simulink library "motorAndLoadSFunLib"  (R2019a)
settings: Solver=ode45  StartTime=0.0  StopTime=10.0  RelTol=1e-3  EnableMultiTasking=on
settings Model: Creator=The MathWorks, Inc.  LastModifiedBy=The MathWorks, Inc.
settings DataIOCC: LimitDataPoints=on  SaveFormat=Array  ReturnWorkspaceOutputs=off
settings OptimizationCC: ExpressionDepthLimit=2147483647  LifeSpan=inf
settings DebuggingCC: UnderspecifiedInitializationDetection=Classic  MergeDetectMultiDrivingBlocksExec=none  SolverPrmCheckMsg=warning  AllowSymbolicDim=off  StateNameClashWarn=warning  SFUnexpectedBacktrackingDiag=warning  SFNoUnconditionalDefaultTransitionDiag=warning  SFExecutionAtInitializationDiag=none  ArithmeticOperatorsInVariantConditions=warning
settings HardwareCC: ProdBitPerPointer=32  ProdBitPerSizeT=32  ProdBitPerPtrDiffT=32  ProdLargestAtomicFloat=None  ProdIntDivRoundTo=Undefined  ProdEndianess=Unspecified  ProdWordSize=32  ProdHWDeviceType=32-bit Generic
settings ModelReferenceCC: PropagateSignalLabelsOutOfModel=off
settings SFSimCC: SimUseLocalCustomCode=off
settings RTWCC: RTWUseLocalCustomCode=off
settings CodeAppCC: StateflowObjectComments=on
settings GRTTargetCC: TargetLangStandard=C89/C90 (ANSI)  GeneratePreprocessorConditionals=Disable all
settings ConfigComp: CovMetricSettings=dw  CovHtmlReporting=on  CovSaveCumulativeToWorkspaceVar=on  CovSaveSingleToWorkspaceVar=on  CovExternalEMLEnable=off  CovSFcnEnable=off

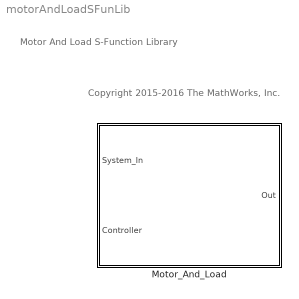
== system motorAndLoadSFunLib ==
  note: Motor And Load S-Function Library
  note: Copyright 2015-2016 The MathWorks, Inc.
  Motor_And_Load : Subsystem
      mask help:
      | This block is provided for users that do not have SimPowerSystems installed but still want to explore the system level simulation without changing motor and load parameter data.
      |
      | This block provides equiavelent functionality to the example library motorAndLoadSimPowerSystemsLib using the default data values included with this example. If you modify data associated with this example, they will NOT be reflected in this block.
      |
      | Please install SimPowerSystems to explore the effects of changing motor and load data including: pmsm, inverter, encoder, and adc values associated with this model.
      mask Display: image('focZynqMotorAndLoadMask.png');

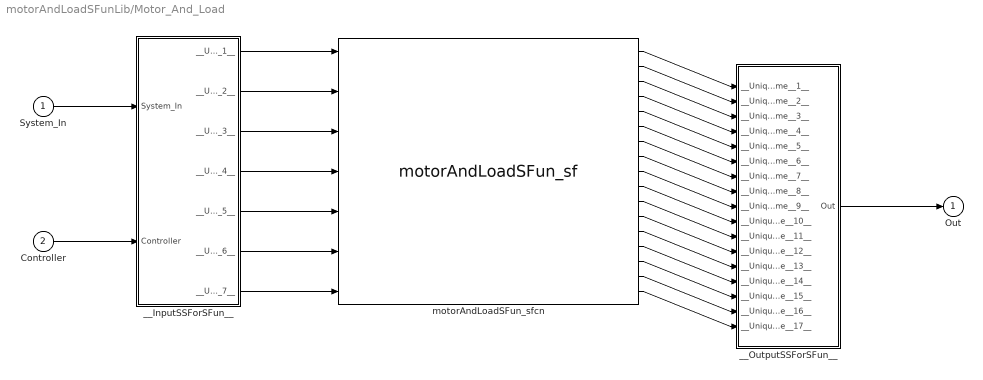
== system motorAndLoadSFunLib/Motor_And_Load ==
  System_In : Inport
  Controller : Inport  Port=2
  __InputSSForSFun__ : Subsystem
  __OutputSSForSFun__ : Subsystem
  motorAndLoadSFun_sfcn : S-Function  FunctionName=motorAndLoadSFun_sf  SFunctionModules=""  SFunctionDeploymentMode=off  EnableBusSupport=off  mask{rtw_sf_name=motorAndLoadSFun_sf, showVar=off}
      mask prompts: rtw_sf_name "Simulink:masks:GenSFuncName_MP"; showVar "Simulink:masks:GenSFuncShowModuleList_MP"
      mask help: Simulink:masks:GenSFuncDesc_MD
      mask init:
      | displist = '';
      | if ~strcmp(get_param(gcb, 'FunctionName'), rtw_sf_name);
      |   set_param(gcb, 'FunctionName', rtw_sf_name);
      | end
      | % Check if we are generating code
      | rtw_mode = false;
      | if strcmpi(get_param(bdroot(gcb),'SimulationStatus'),'Initializing')
      | 	rtw_mode = strcmpi(get_param(bdroot(gcb),'BuildingRTWCode'),'on') && ...
      | 		~strcmpi(get_param(bdroot(gcb),'TargetStyle'),'SimulationTarget');
      | end
      | if showVar || rtw_mode
      | 	if exist('rtwsfunc') == 2 | exist('rtwsfunc') == 6
      | 		tmplist = rtwsfunc(rtw_sf_name,gcb);
      | 		tmplist = DAStudio.message('Simulink:masks:GenSFuncListOfModules_IC', tmplist);
      | 	elseif showVar
      | 		tmplist1 = DAStudio.message('Simulink:masks:GenSFuncListOfModules_IC', '');
      |         tmplist2 = DAStudio.message('Simulink:masks:GenSFuncNotLicensed_IC');
      |         tmplist = [tmplist1 tmplist2];
      |  	end
      | end
      | if showVar
      |   displist = tmplist;
      | end
      settings: CopyFcn=|
      | if ~strcmp(get_param(gcb,'Linkstatus'),'none') && ...
      | ~strcmp(get_param(gcb,'Linkstatus'),'implicit')
      |   set_param(gcb,'LinkStatus','none');
      | end
      mask Help: eval('feval(''rtwprivate'',''rtwhelpview'',''rtw_sfcn_block'')');
      mask Display:
      | port_label('input',1,'motorOn');
      | port_label('input',2,'commandType');
      | port_label('input',3,'velocityCommand');
      | port_label('input',4,'dynoLoadDutyCycle');
      | port_label('input',5,'controllerMode');
      | port_label('input',6,'inverterEnable');
      | port_label('input',7,'pwmCompare');
      | port_label('output',1,'controllerModeb');
      | port_label('output',2,'inverterEnableb');
      | port_label('output',3,'pwmCompareb');
      | port_label('output',4,'phaseVoltage');
      | port_label('output',5,'phaseCurrentA');
      | port_label('output',6,'phaseCurrentB');
      | port_label('output',7,'phaseCurrentC');
      | port_label('output',8,'directCurrent');
      | port_label('output',9,'quadratureCurrent');
      | port_label('output',10,'electromagneticTorque');
      | port_label('output',11,'rotorPosition');
      | port_label('output',12,'electricalPosition');
      | port_label('output',13,'rotorVelocity');
      | port_label('output',14,'electricalVelocity');
      | port_label('output',15,'adcCount');
      | port_label('output',16,'encoderIndexFound');
      | port_label('output',17,'encoderCount');
  Out : Outport
  wires:
  __OutputSSForSFun__/1(Out) -> Out/1
  motorAndLoadSFun_sfcn/17 -> __OutputSSForSFun__/17(__UniqueInportName__17__)
  motorAndLoadSFun_sfcn/16 -> __OutputSSForSFun__/16(__UniqueInportName__16__)
  motorAndLoadSFun_sfcn/15 -> __OutputSSForSFun__/15(__UniqueInportName__15__)
  motorAndLoadSFun_sfcn/14 -> __OutputSSForSFun__/14(__UniqueInportName__14__)
  motorAndLoadSFun_sfcn/13 -> __OutputSSForSFun__/13(__UniqueInportName__13__)
  motorAndLoadSFun_sfcn/12 -> __OutputSSForSFun__/12(__UniqueInportName__12__)
  motorAndLoadSFun_sfcn/11 -> __OutputSSForSFun__/11(__UniqueInportName__11__)
  motorAndLoadSFun_sfcn/10 -> __OutputSSForSFun__/10(__UniqueInportName__10__)
  motorAndLoadSFun_sfcn/9 -> __OutputSSForSFun__/9(__UniqueInportName__9__)
  motorAndLoadSFun_sfcn/8 -> __OutputSSForSFun__/8(__UniqueInportName__8__)
  motorAndLoadSFun_sfcn/7 -> __OutputSSForSFun__/7(__UniqueInportName__7__)
  motorAndLoadSFun_sfcn/6 -> __OutputSSForSFun__/6(__UniqueInportName__6__)
  motorAndLoadSFun_sfcn/5 -> __OutputSSForSFun__/5(__UniqueInportName__5__)
  motorAndLoadSFun_sfcn/4 -> __OutputSSForSFun__/4(__UniqueInportName__4__)
  motorAndLoadSFun_sfcn/3 -> __OutputSSForSFun__/3(__UniqueInportName__3__)
  motorAndLoadSFun_sfcn/2 -> __OutputSSForSFun__/2(__UniqueInportName__2__)
  motorAndLoadSFun_sfcn/1 -> __OutputSSForSFun__/1(__UniqueInportName__1__)
  __InputSSForSFun__/7(__UniqueOutportName__7__) -> motorAndLoadSFun_sfcn/7
  __InputSSForSFun__/6(__UniqueOutportName__6__) -> motorAndLoadSFun_sfcn/6
  __InputSSForSFun__/5(__UniqueOutportName__5__) -> motorAndLoadSFun_sfcn/5
  __InputSSForSFun__/4(__UniqueOutportName__4__) -> motorAndLoadSFun_sfcn/4
  __InputSSForSFun__/3(__UniqueOutportName__3__) -> motorAndLoadSFun_sfcn/3
  __InputSSForSFun__/2(__UniqueOutportName__2__) -> motorAndLoadSFun_sfcn/2
  __InputSSForSFun__/1(__UniqueOutportName__1__) -> motorAndLoadSFun_sfcn/1
  Controller/1 -> __InputSSForSFun__/2(Controller)
  System_In/1 -> __InputSSForSFun__/1(System_In)

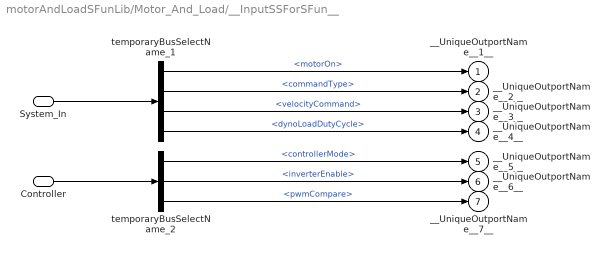
== system motorAndLoadSFunLib/Motor_And_Load/__InputSSForSFun__ ==
  System_In : Inport
  Controller : Inport  Port=2
  temporaryBusSelectName_1 : BusSelector  OutputSignals=motorOn,commandType,velocityCommand,dynoLoadDutyCycle
  temporaryBusSelectName_2 : BusSelector  OutputSignals=controllerMode,inverterEnable,pwmCompare
  __UniqueOutportName__1__ : Outport
  __UniqueOutportName__2__ : Outport  Port=2
  __UniqueOutportName__3__ : Outport  Port=3
  __UniqueOutportName__4__ : Outport  Port=4
  __UniqueOutportName__5__ : Outport  Port=5
  __UniqueOutportName__6__ : Outport  Port=6
  __UniqueOutportName__7__ : Outport  Port=7
  wires:
  temporaryBusSelectName_2/3 -> __UniqueOutportName__7__/1  "<pwmCompare>"
  temporaryBusSelectName_2/2 -> __UniqueOutportName__6__/1  "<inverterEnable>"
  temporaryBusSelectName_2/1 -> __UniqueOutportName__5__/1  "<controllerMode>"
  temporaryBusSelectName_1/4 -> __UniqueOutportName__4__/1  "<dynoLoadDutyCycle>"
  temporaryBusSelectName_1/3 -> __UniqueOutportName__3__/1  "<velocityCommand>"
  temporaryBusSelectName_1/2 -> __UniqueOutportName__2__/1  "<commandType>"
  temporaryBusSelectName_1/1 -> __UniqueOutportName__1__/1  "<motorOn>"
  Controller/1 -> temporaryBusSelectName_2/1
  System_In/1 -> temporaryBusSelectName_1/1

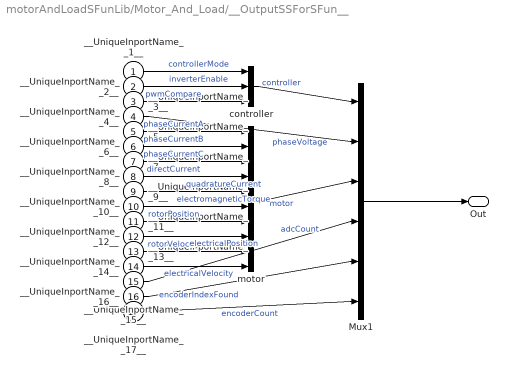
== system motorAndLoadSFunLib/Motor_And_Load/__OutputSSForSFun__ ==
  __UniqueInportName__1__ : Inport
  __UniqueInportName__2__ : Inport  Port=2
  __UniqueInportName__3__ : Inport  Port=3
  __UniqueInportName__4__ : Inport  Port=4
  __UniqueInportName__5__ : Inport  Port=5
  __UniqueInportName__6__ : Inport  Port=6
  __UniqueInportName__7__ : Inport  Port=7
  __UniqueInportName__8__ : Inport  Port=8
  __UniqueInportName__9__ : Inport  Port=9
  __UniqueInportName__10__ : Inport  Port=10
  __UniqueInportName__11__ : Inport  Port=11
  __UniqueInportName__12__ : Inport  Port=12
  __UniqueInportName__13__ : Inport  Port=13
  __UniqueInportName__14__ : Inport  Port=14
  __UniqueInportName__15__ : Inport  Port=15
  __UniqueInportName__16__ : Inport  Port=16
  __UniqueInportName__17__ : Inport  Port=17
  Mux1 : BusCreator  Inputs=6
  controller : BusCreator  Inputs=3
  motor : BusCreator  Inputs=10
  Out : Outport
  wires:
  Mux1/1 -> Out/1
  __UniqueInportName__17__/1 -> Mux1/6  "encoderCount"
  __UniqueInportName__16__/1 -> Mux1/5  "encoderIndexFound"
  __UniqueInportName__15__/1 -> Mux1/4  "adcCount"
  motor/1 -> Mux1/3  "motor"
  __UniqueInportName__4__/1 -> Mux1/2  "phaseVoltage"
  controller/1 -> Mux1/1  "controller"
  __UniqueInportName__14__/1 -> motor/10  "electricalVelocity"
  __UniqueInportName__13__/1 -> motor/9  "rotorVelocity"
  __UniqueInportName__12__/1 -> motor/8  "electricalPosition"
  __UniqueInportName__11__/1 -> motor/7  "rotorPosition"
  __UniqueInportName__10__/1 -> motor/6  "electromagneticTorque"
  __UniqueInportName__9__/1 -> motor/5  "quadratureCurrent"
  __UniqueInportName__8__/1 -> motor/4  "directCurrent"
  __UniqueInportName__7__/1 -> motor/3  "phaseCurrentC"
  __UniqueInportName__6__/1 -> motor/2  "phaseCurrentB"
  __UniqueInportName__5__/1 -> motor/1  "phaseCurrentA"
  __UniqueInportName__3__/1 -> controller/3  "pwmCompare"
  __UniqueInportName__2__/1 -> controller/2  "inverterEnable"
  __UniqueInportName__1__/1 -> controller/1  "controllerMode"
